simulink model "Sim_HDT_Resonant"  (R2025b)
settings: Solver=VariableStepAuto  StartTime=0.0  StopTime=0.3  FixedStep=Ts  RelTol=1e-3
values from neighbouring files (symbols this model uses):
  Ard = blkdiag(Ard1,Ard3,Ard5)    [HDT_Unified_Init.m]
  Brd = [Brd1;Brd3;Brd5]    [HDT_Unified_Init.m]
  Ha = [0 0 1 0 0 0 0 0 0 0 ... (first row only)    [HDT_Unified_Init.m]
  nu = size(Bd,2)    [Sim_HDT.m]
  nxr = size(Brd,1)    [HDT_Unified_Init.m]    (also in Sim_HDT.m)
undefined symbols (not defined in the file or in its folder): A, B, C, Kr, Ku, Kx, Ts, w
settings Model: Creator=dfigueroa  LastModifiedBy=dfigueroa

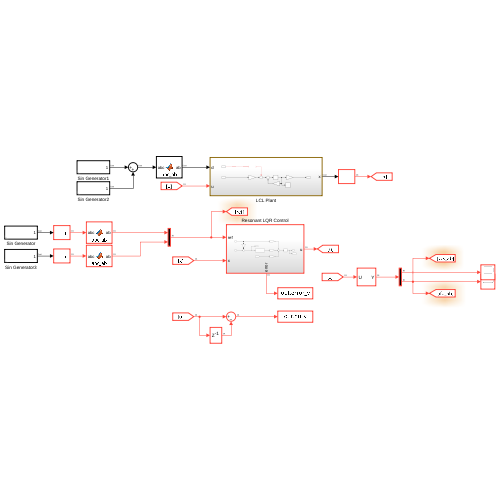
[thumbnail: Simulink's stored preview of the top-level diagram]
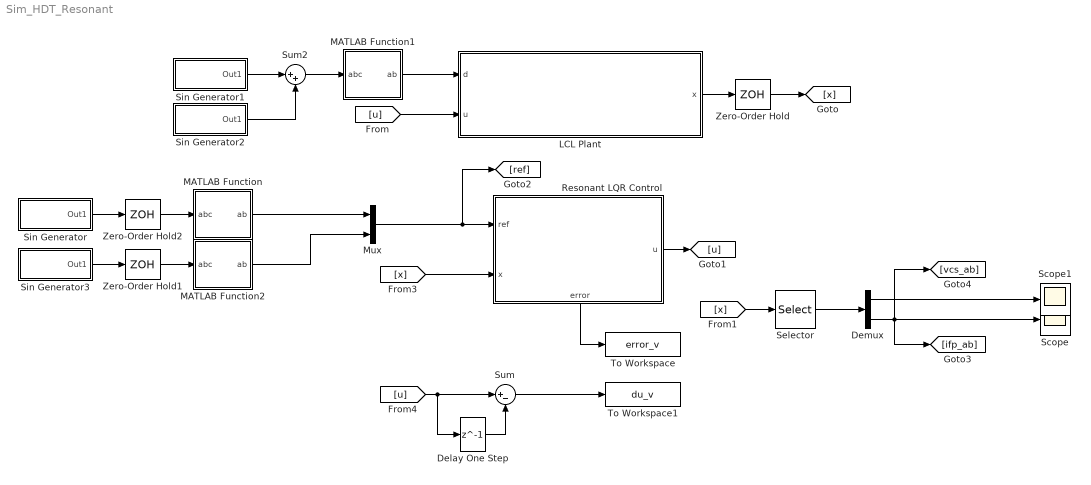
== system Sim_HDT_Resonant ==
  Delay One Step : Delay  DelayLength=1  SampleTime=Ts
  Demux : Demux  Outputs=[2;2]
  LCL Plant : Subsystem
  MATLAB Function : MATLAB Function  TreatAsAtomicUnit=on
  MATLAB Function1 : MATLAB Function  TreatAsAtomicUnit=on
  MATLAB Function2 : MATLAB Function  TreatAsAtomicUnit=on
  Mux : Mux  Inputs=[2;2]
  Resonant LQR Control : Subsystem
      settings: PortSchema="{\"entries\":[{\"content\":{\"sides\":[{\"content\":{\"connectorIds\":[\"In1\",\"In2\"]},\"type\":\"ConnectorPlacement.EquallySpacedRectSide\",\"uuid\":\"99a690ac-3bd0-4f81-b659-f279a9474794\"},{\"content\":{\"connectorIds\":[\"Out1\"],\"side\":\"RIGHT\"},\"type\":\"ConnectorPlacement.EquallySpacedRectSide\",\"uuid\":\"8cc57969-c53c-48c8-8db6-de6ebbedc9fa\"},{\"content\":{\"side\":\"TOP\"},\"type\":\"ConnectorPlacement.EquallySpacedRectSide\",\"uuid\":\"feb69ac5-7da0-4fd7-b564-be03e1a824d1\"},{\"content\":{\"connectorIds\":[\"Out2\"],\"side\":\"BOTTOM\"},\"type\":\"ConnectorPlacement.EquallySpacedRectSide\",\"uuid\":\"e21016e3-b19c-4730-ba77-eca85728fa6b\"}]},\"type\":\"ConnectorPlacement.EquallySpacedConnector\",\"uuid\":\"29586c0e-7c9a-4d19-baa4-f2b2392acca9\"}],\"packageUris\":[\"http://schema.mathworks.com/mf0/Connector/R2020b\"],\"version\":\"1.0\"}"
  Scope : Scope
      settings: ActiveDisplayYMinimum=-5.9626941889516756  ActiveDisplayYMaximum=5.9619361192932505
  Scope1 : Scope
      settings: ActiveDisplayYMinimum=-125.00003514127394  ActiveDisplayYMaximum=125.00003514127394
  Selector : Selector  InputPortWidth=10  IndexOptions=Index vector (dialog)  Indices=[3 4 5 6]  OutputSizes=1
  Sin Generator : Subsystem  mask{w=w, Amp=100, Tset=0.02, Tstep=0.02}
      mask prompts: w "Frequency"; Amp "Reference Amplitude"; Tset "Set Time [s]"; Tstep "Step Time"
  Sin Generator1 : Subsystem  mask{w=w, Amp=0, Tset=0, Tstep=0.1}
      mask prompts: w "Frequency"; Amp "Reference Amplitude"; Tset "Set Time [s]"; Tstep "Step Time"
  Sin Generator2 : Subsystem  mask{w=3*w, Amp=0, Tset=0, Tstep=0.1}
      mask prompts: w "Frequency"; Amp "Reference Amplitude"; Tset "Set Time [s]"; Tstep "Step Time"
  Sin Generator3 : Subsystem  mask{w=w, Amp=5, Tset=0.02, Tstep=0.06}
      mask prompts: w "Frequency"; Amp "Reference Amplitude"; Tset "Set Time [s]"; Tstep "Step Time"
  Sum : Sum  Inputs=|+-
  Sum2 : Sum  Inputs=|++
  To Workspace : ToWorkspace  VariableName=error_v  SampleTime=Ts
  To Workspace1 : ToWorkspace  VariableName=du_v  SampleTime=Ts
  Zero-Order Hold : ZeroOrderHold  SampleTime=Ts
  Zero-Order Hold1 : ZeroOrderHold  SampleTime=Ts
  Zero-Order Hold2 : ZeroOrderHold  SampleTime=Ts
  wires:
  Demux/2 -> [vcs_ab], [ifp_ab], Scope/1
  [x] -> Selector/1
  Zero-Order Hold/1 -> [x]
  Zero-Order Hold2/1 -> MATLAB Function/1(abc)
  LCL Plant/1(x) -> Zero-Order Hold/1
  [u] -> LCL Plant/2(u)
  [x] -> Resonant LQR Control/2(x)
  Resonant LQR Control/1(u) -> [u]
  Sin Generator/1(Out1) -> Zero-Order Hold2/1
  Mux/1 -> [ref], Resonant LQR Control/1(ref)
  [u] -> Delay One Step/1, Sum/1
  Delay One Step/1 -> Sum/2
  Resonant LQR Control/2(error) -> To Workspace/1
  Sin Generator1/1(Out1) -> Sum2/1
  Sum/1 -> To Workspace1/1
  Sum2/1 -> MATLAB Function1/1(abc)
  Demux/1 -> Scope1/1
  MATLAB Function1/1(ab) -> LCL Plant/1(d)
  Sin Generator2/1(Out1) -> Sum2/2
  MATLAB Function/1(ab) -> Mux/1
  Sin Generator3/1(Out1) -> Zero-Order Hold1/1
  Zero-Order Hold1/1 -> MATLAB Function2/1(abc)
  MATLAB Function2/1(ab) -> Mux/2
  Selector/1 -> Demux/1

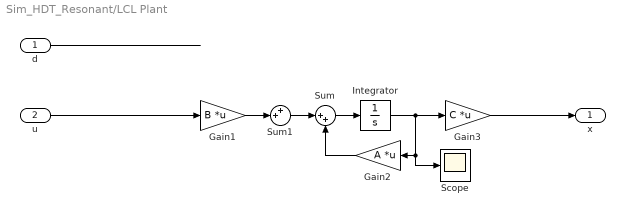
== system Sim_HDT_Resonant/LCL Plant ==
  d : Inport
  u : Inport  Port=2
  Gain1 : Gain  Gain=B  Multiplication=Matrix(K*u)
  Gain2 : Gain  Gain=A  Multiplication=Matrix(K*u)
  Gain3 : Gain  Gain=C  Multiplication=Matrix(K*u)
  Integrator : Integrator
  Scope : Scope
      settings: ActiveDisplayYMinimum=-2.0754804091592516  ActiveDisplayYMaximum=6.2101337392628384  DataLoggingVariableName=ScopeData3
  Sum : Sum  Inputs=|++
  Sum1 : Sum  Inputs=++|
  x : Outport
  wires:
  u/1 -> Gain1/1
  Gain2/1 -> Sum/2
  ? -> Sum1/1
  Sum/1 -> Integrator/1
  Integrator/1 -> Gain3/1, Scope/1, Gain2/1
  d/1 -> ?
  Sum1/1 -> Sum/1
  Gain1/1 -> Sum1/2
  Gain3/1 -> x/1

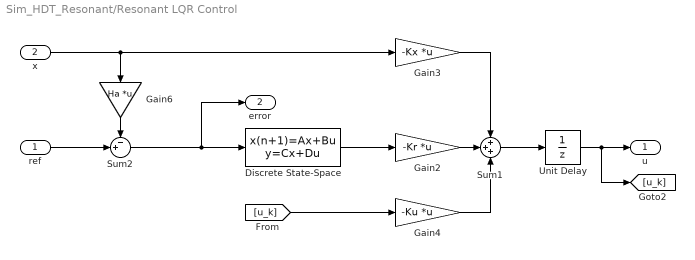
== system Sim_HDT_Resonant/Resonant LQR Control ==
  ref : Inport
  x : Inport  Port=2
  Discrete State-Space : DiscreteStateSpace  A=Ard  B=Brd  C=eye(nxr)  D=zeros(nxr,nu)  SampleTime=Ts
  Gain2 : Gain  Gain=-Kr  Multiplication=Matrix(K*u)
  Gain3 : Gain  Gain=-Kx  Multiplication=Matrix(K*u)
  Gain4 : Gain  Gain=-Ku  Multiplication=Matrix(K*u)
  Gain6 : Gain  Gain=Ha  Multiplication=Matrix(K*u)
  Sum1 : Sum  Inputs=+++
  Sum2 : Sum  Inputs=-+|
  Unit Delay : UnitDelay  SampleTime=Ts  HasFrameUpgradeWarning=on
  u : Outport
  error : Outport  Port=2
  wires:
  x/1 -> Gain6/1, Gain3/1
  Gain6/1 -> Sum2/1
  Unit Delay/1 -> [u_k], u/1
  ref/1 -> Sum2/2
  Gain2/1 -> Sum1/2
  Gain3/1 -> Sum1/1
  Gain4/1 -> Sum1/3
  [u_k] -> Gain4/1
  Sum1/1 -> Unit Delay/1
  Sum2/1 -> error/1, Discrete State-Space/1
  Discrete State-Space/1 -> Gain2/1

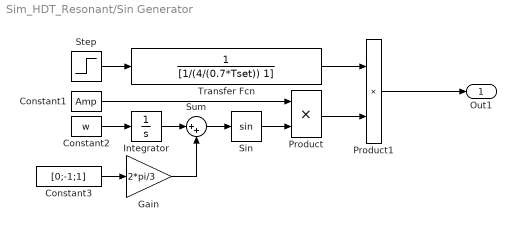
== system Sim_HDT_Resonant/Sin Generator ==
  Constant1 : Constant  Value=Amp
  Constant2 : Constant  Value=w
  Constant3 : Constant  Value=[0;-1;1]
  Gain : Gain  Gain=2*pi/3
  Integrator : Integrator
  Product : Product
  Product1 : Product
  Sin : Trigonometry
  Step : Step  Time=Tstep  SampleTime=0
  Sum : Sum  Inputs=|++
  Transfer Fcn : TransferFcn  Denominator=[1/(4/(0.7*Tset)) 1]
  Out1 : Outport
  wires:
  Sum/1 -> Sin/1
  Transfer Fcn/1 -> Product1/1
  Constant2/1 -> Integrator/1
  Integrator/1 -> Sum/1
  Constant1/1 -> Product/1
  Constant3/1 -> Gain/1
  Product1/1 -> Out1/1
  Gain/1 -> Sum/2
  Step/1 -> Transfer Fcn/1
  Sin/1 -> Product/2
  Product/1 -> Product1/2

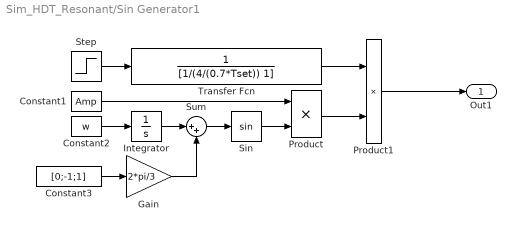
== system Sim_HDT_Resonant/Sin Generator1 ==
  Constant1 : Constant  Value=Amp
  Constant2 : Constant  Value=w
  Constant3 : Constant  Value=[0;-1;1]
  Gain : Gain  Gain=2*pi/3
  Integrator : Integrator
  Product : Product
  Product1 : Product
  Sin : Trigonometry
  Step : Step  Time=Tstep  SampleTime=0
  Sum : Sum  Inputs=|++
  Transfer Fcn : TransferFcn  Denominator=[1/(4/(0.7*Tset)) 1]
  Out1 : Outport
  wires:
  Product/1 -> Product1/2
  Sin/1 -> Product/2
  Step/1 -> Transfer Fcn/1
  Gain/1 -> Sum/2
  Product1/1 -> Out1/1
  Constant3/1 -> Gain/1
  Constant1/1 -> Product/1
  Integrator/1 -> Sum/1
  Constant2/1 -> Integrator/1
  Transfer Fcn/1 -> Product1/1
  Sum/1 -> Sin/1

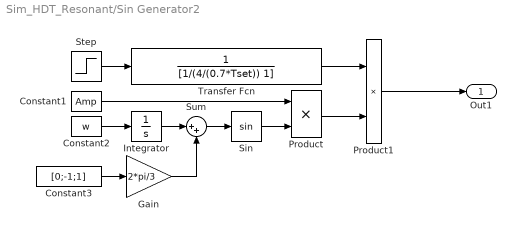
== system Sim_HDT_Resonant/Sin Generator2 ==
  Constant1 : Constant  Value=Amp
  Constant2 : Constant  Value=w
  Constant3 : Constant  Value=[0;-1;1]
  Gain : Gain  Gain=2*pi/3
  Integrator : Integrator
  Product : Product
  Product1 : Product
  Sin : Trigonometry
  Step : Step  Time=Tstep  SampleTime=0
  Sum : Sum  Inputs=|++
  Transfer Fcn : TransferFcn  Denominator=[1/(4/(0.7*Tset)) 1]
  Out1 : Outport
  wires:
  Sum/1 -> Sin/1
  Transfer Fcn/1 -> Product1/1
  Constant2/1 -> Integrator/1
  Integrator/1 -> Sum/1
  Constant1/1 -> Product/1
  Constant3/1 -> Gain/1
  Product1/1 -> Out1/1
  Gain/1 -> Sum/2
  Step/1 -> Transfer Fcn/1
  Sin/1 -> Product/2
  Product/1 -> Product1/2

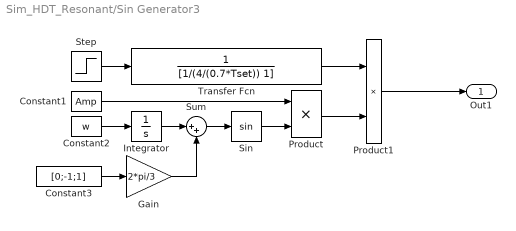
== system Sim_HDT_Resonant/Sin Generator3 ==
  Constant1 : Constant  Value=Amp
  Constant2 : Constant  Value=w
  Constant3 : Constant  Value=[0;-1;1]
  Gain : Gain  Gain=2*pi/3
  Integrator : Integrator
  Product : Product
  Product1 : Product
  Sin : Trigonometry
  Step : Step  Time=Tstep  SampleTime=0
  Sum : Sum  Inputs=|++
  Transfer Fcn : TransferFcn  Denominator=[1/(4/(0.7*Tset)) 1]
  Out1 : Outport
  wires:
  Product/1 -> Product1/2
  Sin/1 -> Product/2
  Step/1 -> Transfer Fcn/1
  Gain/1 -> Sum/2
  Product1/1 -> Out1/1
  Constant3/1 -> Gain/1
  Constant1/1 -> Product/1
  Integrator/1 -> Sum/1
  Constant2/1 -> Integrator/1
  Transfer Fcn/1 -> Product1/1
  Sum/1 -> Sin/1

== matlab function Sim_HDT_Resonant/MATLAB Function ==
  data: abc input; ab output
function ab = abc_ab(abc)
    alpha = (2*abc(1) - abc(2) - abc(3))/3;
    beta = (abc(2) - abc(3))/sqrt(3);
ab = [alpha;beta];

== matlab function Sim_HDT_Resonant/MATLAB Function2 ==
  data: abc input; ab output
function ab = abc_ab(abc)
    alpha = (2*abc(1) - abc(2) - abc(3))/3;
    beta = (abc(2) - abc(3))/sqrt(3);
ab = [alpha;beta];

== matlab function Sim_HDT_Resonant/MATLAB Function1 ==
  data: abc input; ab output
function ab = abc_ab(abc)
    alpha = (2*abc(1) - abc(2) - abc(3))/3;
    beta = (abc(2) - abc(3))/sqrt(3);
ab = [alpha;beta];
